simulink model "pld16x8"  (R2020a)
settings: Solver=VariableStepAuto  StartTime=0.0  StopTime=10.0  RelTol=1e-3
settings Model: Creator=kishan  LastModifiedBy=kishan

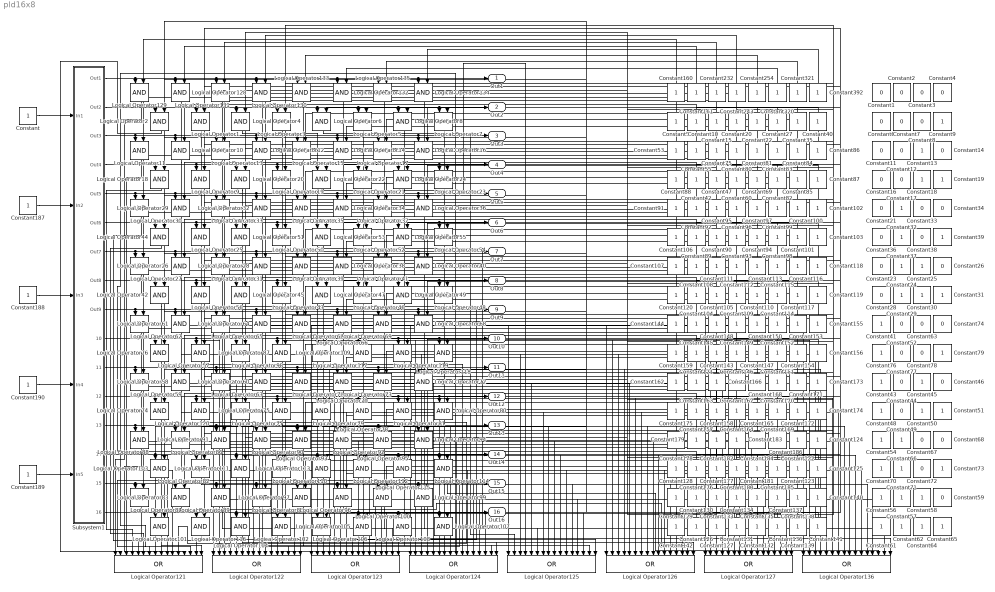
== system pld16x8 ==
  Constant{,5,9..10,13,15,18..20,22,24..25,27,29..32,35,37,39..43,45,47..48,50..51,53..58,60..62,64..66,69..71,73,75..76,79..190,232,243,254,320..321,392} (165 alike) : Constant
  Constant{1..4,6..8,11..12,14,16..17,21,23,26,28,33..34,36,38,44,46,49,52,59,63,67..68,72,74,77..78} (32 alike) : Constant  Value=0
  Logical Operator{1..120,128..135} (128 alike) : Logic  AllPortsSameDT=off  OutDataTypeStr=boolean
  Logical Operator{121..127,136} (8 alike) : Logic  Operator=OR  Inputs=16  AllPortsSameDT=off  OutDataTypeStr=boolean
  Subsystem1 : Subsystem
  Out1 : Outport
  Out2 : Outport  Port=2
  Out3 : Outport  Port=3
  Out4 : Outport  Port=4
  Out5 : Outport  Port=5
  Out6 : Outport  Port=6
  Out7 : Outport  Port=7
  Out8 : Outport  Port=8
  Out9 : Outport  Port=9
  Out10 : Outport  Port=10
  Out11 : Outport  Port=11
  Out12 : Outport  Port=12
  Out13 : Outport  Port=13
  Out14 : Outport  Port=14
  Out15 : Outport  Port=15
  Out16 : Outport  Port=16
  wires:
  Subsystem1/1(Out1) -> Out1/1, Logical Operator134/1, Logical Operator135/1, Logical Operator132/1, Logical Operator133/1, Logical Operator130/1, Logical Operator131/1, Logical Operator128/1, Logical Operator129/1
  Subsystem1/2(Out2) -> Out2/1, Logical Operator7/1, Logical Operator8/1, Logical Operator5/1, Logical Operator6/1, Logical Operator3/1, Logical Operator4/1, Logical Operator1/1, Logical Operator2/1
  Constant160/1 -> Logical Operator129/2
  Constant161/1 -> Logical Operator128/2
  Constant232/1 -> Logical Operator131/2
  Constant243/1 -> Logical Operator130/2
  Constant254/1 -> Logical Operator133/2
  Constant320/1 -> Logical Operator132/2
  Constant321/1 -> Logical Operator135/2
  Constant392/1 -> Logical Operator134/2
  Constant5/1 -> Logical Operator2/2
  Constant10/1 -> Logical Operator1/2
  Constant15/1 -> Logical Operator4/2
  Constant20/1 -> Logical Operator3/2
  Constant22/1 -> Logical Operator6/2
  Constant27/1 -> Logical Operator5/2
  Constant35/1 -> Logical Operator8/2
  Constant40/1 -> Logical Operator7/2
  Constant83/1 -> Logical Operator14/2
  Constant88/1 -> Logical Operator18/2
  Constant81/1 -> Logical Operator15/2
  Constant60/1 -> Logical Operator19/2
  Subsystem1/4(Out4) -> Out4/1, Logical Operator23/1, Logical Operator24/1, Logical Operator21/1, Logical Operator22/1, Logical Operator19/1, Logical Operator20/1, Logical Operator9/1, Logical Operator18/1
  Constant42/1 -> Logical Operator9/2
  Constant82/1 -> Logical Operator21/2
  Constant75/1 -> Logical Operator13/2
  Constant47/1 -> Logical Operator20/2
  Constant53/1 -> Logical Operator11/2
  Constant69/1 -> Logical Operator22/2
  Constant85/1 -> Logical Operator24/2
  Constant80/1 -> Logical Operator12/2
  Subsystem1/3(Out3) -> Out3/1, Logical Operator16/1, Logical Operator17/1, Logical Operator14/1, Logical Operator15/1, Logical Operator12/1, Logical Operator13/1, Logical Operator10/1, Logical Operator11/1
  Constant86/1 -> Logical Operator16/2
  Constant84/1 -> Logical Operator17/2
  Constant87/1 -> Logical Operator23/2
  Constant55/1 -> Logical Operator10/2
  Constant99/1 -> Logical Operator34/2
  Constant108/1 -> Logical Operator26/2
  Constant116/1 -> Logical Operator41/2
  Constant119/1 -> Logical Operator48/2
  Constant97/1 -> Logical Operator35/2
  Constant106/1 -> Logical Operator44/2
  Constant113/1 -> Logical Operator39/2
  Constant91/1 -> Logical Operator30/2
  Constant114/1 -> Logical Operator46/2
  Constant112/1 -> Logical Operator28/2
  Subsystem1/8(Out8) -> Out8/1, Logical Operator48/1, Logical Operator49/1, Logical Operator46/1, Logical Operator47/1, Logical Operator43/1, Logical Operator45/1, Logical Operator56/1, Logical Operator42/1
  Constant89/1 -> Logical Operator25/2
  Constant110/1 -> Logical Operator47/2
  Constant98/1 -> Logical Operator52/2
  Constant101/1 -> Logical Operator55/2
  Constant90/1 -> Logical Operator51/2
  Constant94/1 -> Logical Operator53/2
  Subsystem1/6(Out6) -> Out6/1, Logical Operator54/1, Logical Operator55/1, Logical Operator52/1, Logical Operator53/1, Logical Operator50/1, Logical Operator51/1, Logical Operator25/1, Logical Operator44/1
  Constant104/1 -> Logical Operator56/2
  Constant109/1 -> Logical Operator43/2
  Constant115/1 -> Logical Operator38/2
  Constant120/1 -> Logical Operator42/2
  Constant111/1 -> Logical Operator31/2
  Constant93/1 -> Logical Operator50/2
  Constant96/1 -> Logical Operator32/2
  Subsystem1/7(Out7) -> Out7/1, Logical Operator40/1, Logical Operator41/1, Logical Operator38/1, Logical Operator39/1, Logical Operator28/1, Logical Operator31/1, Logical Operator26/1, Logical Operator27/1
  Constant105/1 -> Logical Operator45/2
  Constant95/1 -> Logical Operator33/2
  Subsystem1/5(Out5) -> Out5/1, Logical Operator36/1, Logical Operator37/1, Logical Operator34/1, Logical Operator35/1, Logical Operator32/1, Logical Operator33/1, Logical Operator29/1, Logical Operator30/1
  Constant102/1 -> Logical Operator36/2
  Constant100/1 -> Logical Operator37/2
  Constant117/1 -> Logical Operator49/2
  Constant107/1 -> Logical Operator27/2
  Constant118/1 -> Logical Operator40/2
  Constant103/1 -> Logical Operator54/2
  Constant92/1 -> Logical Operator29/2
  Constant152/1 -> Logical Operator66/2
  Constant169/1 -> Logical Operator78/2
  Constant167/1 -> Logical Operator60/2
  Constant174/1 -> Logical Operator80/2
  Constant148/1 -> Logical Operator65/2
  Constant159/1 -> Logical Operator76/2
  Constant165/1 -> Logical Operator79/2
  Constant170/1 -> Logical Operator70/2
  Constant156/1 -> Logical Operator118/2
  Subsystem1/16(Out16) -> Out16/1, Logical Operator107/1, Logical Operator108/1, Logical Operator105/1, Logical Operator106/1, Logical Operator102/1, Logical Operator104/1, Logical Operator116/1, Logical Operator101/1
  Subsystem1/15(Out15) -> Out15/1, Logical Operator99/1, Logical Operator100/1, Logical Operator96/1, Logical Operator97/1, Logical Operator85/1, Logical Operator89/1, Logical Operator83/1, Logical Operator84/1
  Constant150/1 -> Logical Operator67/2
  Constant147/1 -> Logical Operator117/2
  Constant128/1 -> Logical Operator103/2
  Constant162/1 -> Logical Operator59/2
  Constant132/1 -> Logical Operator106/2
  Constant157/1 -> Logical Operator120/2
  Constant186/1 -> Logical Operator92/2
  Constant176/1 -> Logical Operator82/2
  Constant126/1 -> Logical Operator116/2
  Constant133/1 -> Logical Operator89/2
  Subsystem1/13(Out13) -> Out13/1, Logical Operator94/1, Logical Operator95/1, Logical Operator92/1, Logical Operator93/1, Logical Operator90/1, Logical Operator91/1, Logical Operator86/1, Logical Operator88/1
  Constant151/1 -> Logical Operator109/2
  Constant154/1 -> Logical Operator119/2
  Constant177/1 -> Logical Operator111/2
  Constant144/1 -> Logical Operator62/2
  Constant164/1 -> Logical Operator75/2
  Constant134/1 -> Logical Operator85/2
  Constant155/1 -> Logical Operator68/2
  Constant149/1 -> Logical Operator64/2
  Subsystem1/12(Out12) -> Out12/1, Logical Operator80/1, Logical Operator81/1, Logical Operator78/1, Logical Operator79/1, Logical Operator75/1, Logical Operator77/1, Logical Operator120/1, Logical Operator74/1
  Constant184/1 -> Logical Operator93/2
  Constant121/1 -> Logical Operator57/2
  Constant138/1 -> Logical Operator100/2
  Subsystem1/14(Out14) -> Out14/1, Logical Operator114/1, Logical Operator115/1, Logical Operator112/1, Logical Operator113/1, Logical Operator110/1, Logical Operator111/1, Logical Operator82/1, Logical Operator103/1
  Constant124/1 -> Logical Operator94/2
  Constant166/1 -> Logical Operator63/2
  Constant145/1 -> Logical Operator61/2
  Constant136/1 -> Logical Operator105/2
  Constant146/1 -> Logical Operator87/2
  Constant122/1 -> Logical Operator95/2
  Constant129/1 -> Logical Operator84/2
  Constant158/1 -> Logical Operator77/2
  Constant182/1 -> Logical Operator91/2
  Constant153/1 -> Logical Operator69/2
  Constant142/1 -> Logical Operator101/2
  Constant178/1 -> Logical Operator88/2
  Constant130/1 -> Logical Operator83/2
  Subsystem1/10(Out10) -> Out10/1, Logical Operator118/1, Logical Operator119/1, Logical Operator109/1, Logical Operator117/1, Logical Operator87/1, Logical Operator98/1, Logical Operator57/1, Logical Operator76/1
  Constant123/1 -> Logical Operator115/2
  Constant125/1 -> Logical Operator114/2
  Subsystem1/9(Out9) -> Out9/1, Logical Operator68/1, Logical Operator69/1, Logical Operator66/1, Logical Operator67/1, Logical Operator64/1, Logical Operator65/1, Logical Operator61/1, Logical Operator62/1
  Constant181/1 -> Logical Operator113/2
  Constant139/1 -> Logical Operator108/2
  Constant135/1 -> Logical Operator97/2
  Subsystem1/11(Out11) -> Out11/1, Logical Operator72/1, Logical Operator73/1, Logical Operator70/1, Logical Operator71/1, Logical Operator60/1, Logical Operator63/1, Logical Operator58/1, Logical Operator59/1
  Constant163/1 -> Logical Operator58/2
  Constant127/1 -> Logical Operator104/2
  Constant143/1 -> Logical Operator98/2
  Constant171/1 -> Logical Operator73/2
  Constant185/1 -> Logical Operator112/2
  Constant141/1 -> Logical Operator107/2
  Constant175/1 -> Logical Operator74/2
  Constant183/1 -> Logical Operator90/2
  Constant179/1 -> Logical Operator86/2
  Constant168/1 -> Logical Operator71/2
  Constant172/1 -> Logical Operator81/2
  Constant173/1 -> Logical Operator72/2
  Constant180/1 -> Logical Operator110/2
  Constant137/1 -> Logical Operator96/2
  Constant140/1 -> Logical Operator99/2
  Constant131/1 -> Logical Operator102/2
  Logical Operator101/1 -> Logical Operator121/16
  Logical Operator84/1 -> Logical Operator121/15
  Logical Operator103/1 -> Logical Operator121/14
  Logical Operator88/1 -> Logical Operator121/13
  Logical Operator74/1 -> Logical Operator121/12
  Logical Operator59/1 -> Logical Operator121/11
  Logical Operator76/1 -> Logical Operator121/10
  Logical Operator62/1 -> Logical Operator121/9
  Logical Operator42/1 -> Logical Operator121/8
  Logical Operator27/1 -> Logical Operator121/7
  Logical Operator44/1 -> Logical Operator121/6
  Logical Operator30/1 -> Logical Operator121/5
  Logical Operator18/1 -> Logical Operator121/4
  Logical Operator11/1 -> Logical Operator121/3
  Logical Operator2/1 -> Logical Operator121/2
  Logical Operator129/1 -> Logical Operator121/1
  Logical Operator116/1 -> Logical Operator122/16
  Logical Operator83/1 -> Logical Operator122/15
  Logical Operator82/1 -> Logical Operator122/14
  Logical Operator86/1 -> Logical Operator122/13
  Logical Operator120/1 -> Logical Operator122/12
  Logical Operator58/1 -> Logical Operator122/11
  Logical Operator57/1 -> Logical Operator122/10
  Logical Operator61/1 -> Logical Operator122/9
  Logical Operator56/1 -> Logical Operator122/8
  Logical Operator26/1 -> Logical Operator122/7
  Logical Operator25/1 -> Logical Operator122/6
  Logical Operator29/1 -> Logical Operator122/5
  Logical Operator9/1 -> Logical Operator122/4
  Logical Operator10/1 -> Logical Operator122/3
  Logical Operator1/1 -> Logical Operator122/2
  Logical Operator128/1 -> Logical Operator122/1
  Logical Operator104/1 -> Logical Operator123/16
  Logical Operator89/1 -> Logical Operator123/15
  Logical Operator111/1 -> Logical Operator123/14
  Logical Operator91/1 -> Logical Operator123/13
  Logical Operator77/1 -> Logical Operator123/12
  Logical Operator63/1 -> Logical Operator123/11
  Logical Operator98/1 -> Logical Operator123/10
  Logical Operator65/1 -> Logical Operator123/9
  Logical Operator45/1 -> Logical Operator123/8
  Logical Operator31/1 -> Logical Operator123/7
  Logical Operator51/1 -> Logical Operator123/6
  Logical Operator33/1 -> Logical Operator123/5
  Logical Operator20/1 -> Logical Operator123/4
  Logical Operator13/1 -> Logical Operator123/3
  Logical Operator4/1 -> Logical Operator123/2
  Logical Operator131/1 -> Logical Operator123/1
  Logical Operator130/1 -> Logical Operator124/1
  Logical Operator3/1 -> Logical Operator124/2
  Logical Operator12/1 -> Logical Operator124/3
  Logical Operator19/1 -> Logical Operator124/4
  Logical Operator32/1 -> Logical Operator124/5
  Logical Operator50/1 -> Logical Operator124/6
  Logical Operator28/1 -> Logical Operator124/7
  Logical Operator43/1 -> Logical Operator124/8
  Logical Operator64/1 -> Logical Operator124/9
  Logical Operator87/1 -> Logical Operator124/10
  Logical Operator60/1 -> Logical Operator124/11
  Logical Operator75/1 -> Logical Operator124/12
  Logical Operator90/1 -> Logical Operator124/13
  Logical Operator110/1 -> Logical Operator124/14
  Logical Operator85/1 -> Logical Operator124/15
  Logical Operator102/1 -> Logical Operator124/16
  Logical Operator106/1 -> Logical Operator125/16
  Logical Operator97/1 -> Logical Operator125/15
  Logical Operator113/1 -> Logical Operator125/14
  Logical Operator93/1 -> Logical Operator125/13
  Logical Operator79/1 -> Logical Operator125/12
  Logical Operator71/1 -> Logical Operator125/11
  Logical Operator117/1 -> Logical Operator125/10
  Logical Operator67/1 -> Logical Operator125/9
  Logical Operator47/1 -> Logical Operator125/8
  Logical Operator39/1 -> Logical Operator125/7
  Logical Operator53/1 -> Logical Operator125/6
  Logical Operator35/1 -> Logical Operator125/5
  Logical Operator133/1 -> Logical Operator125/1
  Logical Operator6/1 -> Logical Operator125/2
  Logical Operator15/1 -> Logical Operator125/3
  Logical Operator22/1 -> Logical Operator125/4
  Logical Operator132/1 -> Logical Operator126/1
  Logical Operator5/1 -> Logical Operator126/2
  Logical Operator14/1 -> Logical Operator126/3
  Logical Operator21/1 -> Logical Operator126/4
  Logical Operator34/1 -> Logical Operator126/5
  Logical Operator52/1 -> Logical Operator126/6
  Logical Operator38/1 -> Logical Operator126/7
  Logical Operator46/1 -> Logical Operator126/8
  Logical Operator66/1 -> Logical Operator126/9
  Logical Operator109/1 -> Logical Operator126/10
  Logical Operator70/1 -> Logical Operator126/11
  Logical Operator78/1 -> Logical Operator126/12
  Logical Operator92/1 -> Logical Operator126/13
  Logical Operator112/1 -> Logical Operator126/14
  Logical Operator96/1 -> Logical Operator126/15
  Logical Operator105/1 -> Logical Operator126/16
  Logical Operator135/1 -> Logical Operator127/1
  Logical Operator8/1 -> Logical Operator127/2
  Logical Operator17/1 -> Logical Operator127/3
  Logical Operator24/1 -> Logical Operator127/4
  Logical Operator37/1 -> Logical Operator127/5
  Logical Operator55/1 -> Logical Operator127/6
  Logical Operator41/1 -> Logical Operator127/7
  Logical Operator49/1 -> Logical Operator127/8
  Logical Operator69/1 -> Logical Operator127/9
  Logical Operator119/1 -> Logical Operator127/10
  Logical Operator73/1 -> Logical Operator127/11
  Logical Operator81/1 -> Logical Operator127/12
  Logical Operator95/1 -> Logical Operator127/13
  Logical Operator115/1 -> Logical Operator127/14
  Logical Operator100/1 -> Logical Operator127/15
  Logical Operator108/1 -> Logical Operator127/16
  Logical Operator134/1 -> Logical Operator136/1
  Logical Operator7/1 -> Logical Operator136/2
  Logical Operator16/1 -> Logical Operator136/3
  Logical Operator23/1 -> Logical Operator136/4
  Logical Operator36/1 -> Logical Operator136/5
  Logical Operator54/1 -> Logical Operator136/6
  Logical Operator40/1 -> Logical Operator136/7
  Logical Operator48/1 -> Logical Operator136/8
  Logical Operator68/1 -> Logical Operator136/9
  Logical Operator118/1 -> Logical Operator136/10
  Logical Operator72/1 -> Logical Operator136/11
  Logical Operator80/1 -> Logical Operator136/12
  Logical Operator94/1 -> Logical Operator136/13
  Logical Operator114/1 -> Logical Operator136/14
  Logical Operator99/1 -> Logical Operator136/15
  Logical Operator107/1 -> Logical Operator136/16
  Constant/1 -> Subsystem1/1(In1)
  Constant187/1 -> Subsystem1/2(In2)
  Constant188/1 -> Subsystem1/3(In3)
  Constant189/1 -> Subsystem1/5(In5)
  Constant190/1 -> Subsystem1/4(In4)

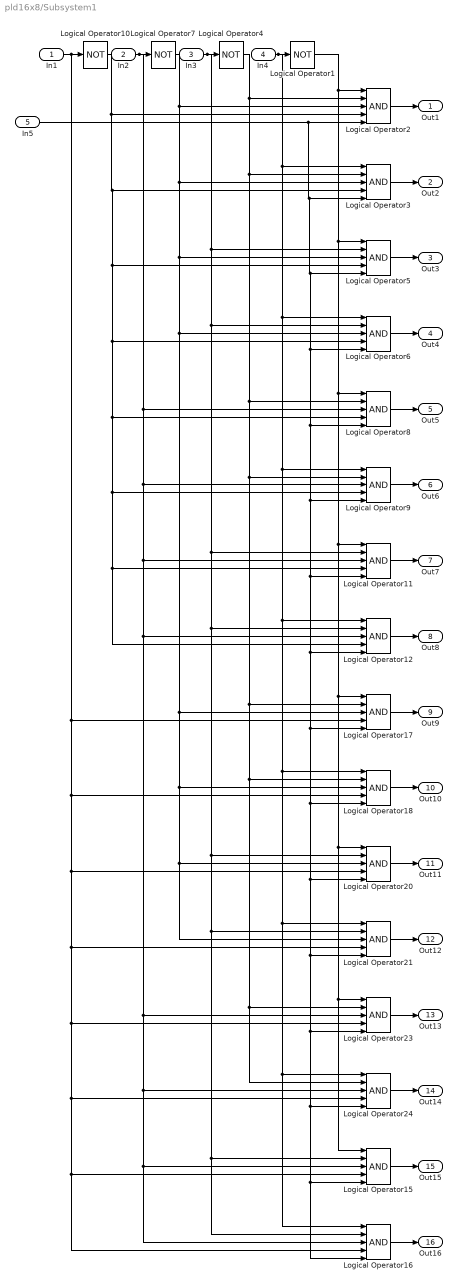
== system pld16x8/Subsystem1 ==
  In1 : Inport
  In2 : Inport  Port=2
  In3 : Inport  Port=3
  In4 : Inport  Port=4
  In5 : Inport  Port=5
  Logical Operator{1,4,7,10} (4 alike) : Logic  Operator=NOT  AllPortsSameDT=off  OutDataTypeStr=boolean
  Logical Operator{2..3,5..6,8..9,11..12,15..18,20..21,23..24} (16 alike) : Logic  Inputs=5  AllPortsSameDT=off  OutDataTypeStr=boolean
  Out1 : Outport
  Out2 : Outport  Port=2
  Out3 : Outport  Port=3
  Out4 : Outport  Port=4
  Out5 : Outport  Port=5
  Out6 : Outport  Port=6
  Out7 : Outport  Port=7
  Out8 : Outport  Port=8
  Out9 : Outport  Port=9
  Out10 : Outport  Port=10
  Out11 : Outport  Port=11
  Out12 : Outport  Port=12
  Out13 : Outport  Port=13
  Out14 : Outport  Port=14
  Out15 : Outport  Port=15
  Out16 : Outport  Port=16
  wires:
  Logical Operator11/1 -> Out7/1
  Logical Operator12/1 -> Out8/1
  Logical Operator18/1 -> Out10/1
  In2/1 -> Logical Operator16/3, Logical Operator15/3, Logical Operator24/3, Logical Operator23/3, Logical Operator12/3, Logical Operator11/3, Logical Operator9/3, Logical Operator8/3, Logical Operator7/1
  In3/1 -> Logical Operator11/2, Logical Operator15/2, Logical Operator16/2, Logical Operator21/2, Logical Operator20/2, Logical Operator12/2, Logical Operator6/2, Logical Operator5/2, Logical Operator4/1
  Logical Operator24/1 -> Out14/1
  In4/1 -> Logical Operator16/1, Logical Operator24/1, Logical Operator21/1, Logical Operator18/1, Logical Operator12/1, Logical Operator9/1, Logical Operator6/1, Logical Operator3/1, Logical Operator1/1
  Logical Operator10/1 -> Logical Operator12/4, Logical Operator11/4, Logical Operator9/4, Logical Operator8/4, Logical Operator6/4, Logical Operator5/4, Logical Operator3/4, Logical Operator2/4
  Logical Operator9/1 -> Out6/1
  In5/1 -> Logical Operator16/5, Logical Operator15/5, Logical Operator24/5, Logical Operator23/5, Logical Operator21/5, Logical Operator20/5, Logical Operator18/5, Logical Operator17/5, Logical Operator12/5, Logical Operator11/5, Logical Operator9/5, Logical Operator8/5, Logical Operator6/5, Logical Operator5/5, Logical Operator3/5, Logical Operator2/5
  Logical Operator5/1 -> Out3/1
  Logical Operator1/1 -> Logical Operator15/1, Logical Operator23/1, Logical Operator20/1, Logical Operator17/1, Logical Operator11/1, Logical Operator8/1, Logical Operator5/1, Logical Operator2/1
  Logical Operator2/1 -> Out1/1
  Logical Operator21/1 -> Out12/1
  Logical Operator8/1 -> Out5/1
  Logical Operator7/1 -> Logical Operator21/3, Logical Operator20/3, Logical Operator18/3, Logical Operator17/3, Logical Operator6/3, Logical Operator5/3, Logical Operator3/3, Logical Operator2/3
  Logical Operator16/1 -> Out16/1
  Logical Operator15/1 -> Out15/1
  In1/1 -> Logical Operator17/4, Logical Operator18/4, Logical Operator20/4, Logical Operator21/4, Logical Operator23/4, Logical Operator24/4, Logical Operator15/4, Logical Operator16/4, Logical Operator10/1
  Logical Operator3/1 -> Out2/1
  Logical Operator20/1 -> Out11/1
  Logical Operator6/1 -> Out4/1
  Logical Operator23/1 -> Out13/1
  Logical Operator4/1 -> Logical Operator24/2, Logical Operator23/2, Logical Operator18/2, Logical Operator17/2, Logical Operator9/2, Logical Operator8/2, Logical Operator3/2, Logical Operator2/2
  Logical Operator17/1 -> Out9/1
